simulink model "EE406_EXP7"  (R2021b)
settings: Solver=FixedStepAuto  StartTime=0.0  StopTime=10.0  FixedStep=0.001  RelTol=1e-3
libraries: slpidlib x1
settings Model: Creator=Powerlab  LastModifiedBy=Powerlab

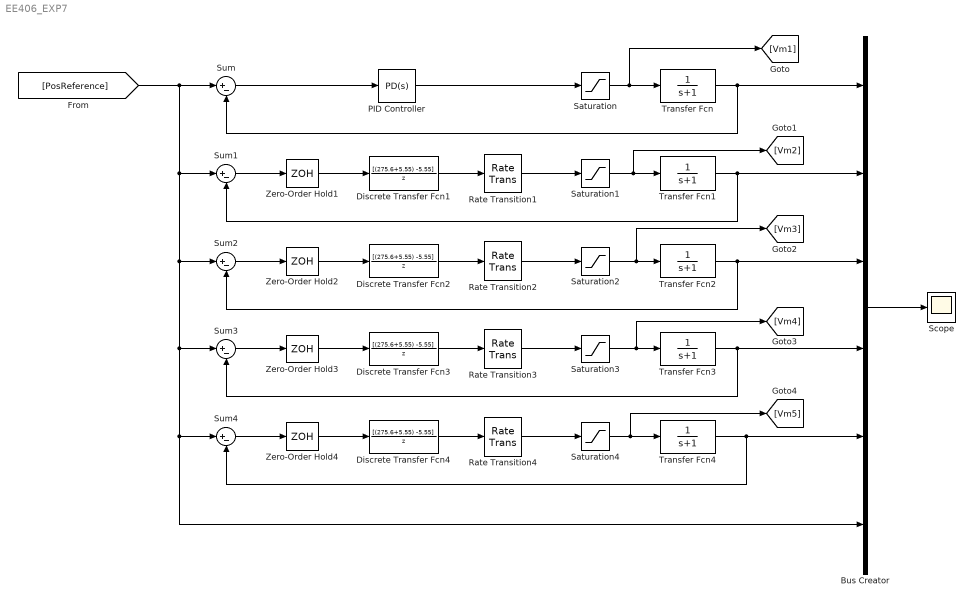
== system EE406_EXP7 ==
  Bus Creator : BusCreator  Inputs=6
  Discrete Transfer Fcn{1..4} (4 alike) : DiscreteTransferFcn  Numerator=[(275.6+5.55) -5.55]  Denominator=[1 0]
  PID Controller : slpidlib/PID Controller  Controller=PD  Form=Parallel  TimeDomain=Continuous-time  UseExternalTs=off  SampleTime=-1  IntegratorMethod=Forward Euler  FilterMethod=Forward Euler  ControllerParametersSource=internal  P=275.6  I=1  D=5.55  UseFilter=on  N=1  TunerSelectOption=Transfer Function Based (PID Tuner App)  InitialConditionSource=internal  InitialConditionForIntegrator=0  InitialConditionForFilter=0  DifferentiatorICPrevScaledInput=0  ExternalReset=none  TrackingMode=off  Kt=1  LimitOutput=off  SatLimitsSource=internal  UpperSaturationLimit=inf  LowerSaturationLimit=-inf  LinearizeAsGain=on  AntiWindupMode=none  Kb=1  POutMin=[]  POutMax=[]  IOutMin=[]  IOutMax=[]  DOutMin=[]  DOutMax=[]  NOutMin=[]  NOutMax=[]  SumOutMin=[]  SumOutMax=[]  SaturationOutMin=[]  SaturationOutMax=[]  PParamMin=[]  PParamMax=[]  IParamMin=[]  IParamMax=[]  DParamMin=[]  DParamMax=[]  NParamMin=[]  NParamMax=[]  KbParamMin=[]  KbParamMax=[]  KtParamMin=[]  KtParamMax=[]  KbOutMin=[]  KbOutMax=[]  KtOutMin=[]  KtOutMax=[]  IntegratorOutMin=[]  IntegratorOutMax=[]  FilterOutMin=[]  FilterOutMax=[]  SumI1OutMin=[]  SumI1OutMax=[]  SumI2OutMin=[]  SumI2OutMax=[]  SumI3OutMin=[]  SumI3OutMax=[]  SumI4OutMin=[]  SumI4OutMax=[]  SumDOutMin=[]  SumDOutMax=[]  DifferentiatorOutMin=[]  DifferentiatorOutMax=[]  FilterDiffOutCoefMin=[]  FilterDiffOutCoefMax=[]  ReciprocalOutMin=[]  ReciprocalOutMax=[]  SumDenOutMin=[]  SumDenOutMax=[]  SumNumOutMin=[]  SumNumOutMax=[]  DivideOutMin=[]  DivideOutMax=[]  UdiffTsProdOutMin=[]  UdiffTsProdOutMax=[]  NTsProdOutMin=[]  NTsProdOutMax=[]  UintegralTsProdOutMin=[]  UintegralTsProdOutMax=[]  UngainTsProdOutMin=[]  UngainTsProdOutMax=[]  IntegratorContinuousStateAttributes=''  IntegratorStateMustResolveToSignalObject=off  IntegratorRTWStateStorageClass=Auto  FilterContinuousStateAttributes=''  FilterStateMustResolveToSignalObject=off  FilterRTWStateStorageClass=Auto  ParallelPVariant=InternalParameters  IdealPVariant=Disabled  IVariant=Disabled  DVariant=InternalParameters  IntegratorVariant=Disabled  SatVariant=Disabled  AWVariant=Disabled  PCopyVariant=Disabled  TRVariant=Disabled  FdbkBlocksVariant=Forward  IdealPFdbkVariant=Disabled  SatFdbkVariant=Disabled  DerivativeFilterVariant=ContFilter  NVariant=InternalParameters  NCopyVariant=Disabled  FilterICVariant=InternalICsFilter  IntegratorICVariant=Disabled  ExternalResetVariant=Disabled  TRSumVariant=Passthrough  SumFdbkVariant=Disabled  SumVariant=Sum_PD  TsampFilterVariant=InternalTs  TsampNgainVariant=Passthrough  TsampIntegralVariant=Disabled_SignalSpec  ExternalSaturationOutDataTypeStr=Inherit: Same as second input
  Rate Transition{1..4} (4 alike) : RateTransition  OutPortSampleTime=0.001
  Saturation{,1..4} (5 alike) : Saturate  UpperLimit=13  LowerLimit=-13
  Scope : Scope
  Sum{,1..4} (5 alike) : Sum  Inputs=|+-
  Transfer Fcn{,1..4} (5 alike) : TransferFcn  Denominator=[1 1]
  Zero-Order Hold1 : ZeroOrderHold  SampleTime=1/500
  Zero-Order Hold2 : ZeroOrderHold  SampleTime=1/100
  Zero-Order Hold3 : ZeroOrderHold  SampleTime=1/50
  Zero-Order Hold4 : ZeroOrderHold  SampleTime=1/10
  wires:
  PID Controller/1 -> Saturation/1
  Saturation/1 -> [Vm1], Transfer Fcn/1
  Sum/1 -> PID Controller/1
  Transfer Fcn/1 -> Sum/2, Bus Creator/1
  Transfer Fcn1/1 -> Sum1/2, Bus Creator/2
  Discrete Transfer Fcn1/1 -> Rate Transition1/1
  Sum1/1 -> Zero-Order Hold1/1
  Rate Transition1/1 -> Saturation1/1
  Zero-Order Hold1/1 -> Discrete Transfer Fcn1/1
  Saturation1/1 -> [Vm2], Transfer Fcn1/1
  Transfer Fcn2/1 -> Sum2/2, Bus Creator/3
  Discrete Transfer Fcn2/1 -> Rate Transition2/1
  Sum2/1 -> Zero-Order Hold2/1
  Rate Transition2/1 -> Saturation2/1
  Zero-Order Hold2/1 -> Discrete Transfer Fcn2/1
  Saturation2/1 -> [Vm3], Transfer Fcn2/1
  Transfer Fcn3/1 -> Sum3/2, Bus Creator/4
  Discrete Transfer Fcn3/1 -> Rate Transition3/1
  Sum3/1 -> Zero-Order Hold3/1
  Rate Transition3/1 -> Saturation3/1
  Zero-Order Hold3/1 -> Discrete Transfer Fcn3/1
  Saturation3/1 -> [Vm4], Transfer Fcn3/1
  Transfer Fcn4/1 -> Sum4/2, Bus Creator/5
  Discrete Transfer Fcn4/1 -> Rate Transition4/1
  Sum4/1 -> Zero-Order Hold4/1
  Rate Transition4/1 -> Saturation4/1
  Zero-Order Hold4/1 -> Discrete Transfer Fcn4/1
  Saturation4/1 -> [Vm5], Transfer Fcn4/1
  [PosReference] -> Sum4/1, Bus Creator/6, Sum3/1, Sum2/1, Sum1/1, Sum/1
  Bus Creator/1 -> Scope/1
